simulink model "Foc_model_Matlab"  (R2024b)
settings: Solver=FixedStepDiscrete  StartTime=0.0  StopTime=5  FixedStep=Ts_simulink  RelTol=1e-3  EnableMultiTasking=on
PreLoadFcn:
  | mcb_pmsm_foc_hall_S32K144EVB_data;
InitFcn:
  | mbd_s32k_consistency_checks(bdroot(gcs));
model workspace (MAT data in the model file):
  IDC_OVERCURRENT : Simulink.Parameter (value not decoded)
  VDC_OVERVOLTAGE : Simulink.Parameter (value not decoded)
  VDC_UNDERVOLTAGE : Simulink.Parameter (value not decoded)
values from neighbouring files (symbols this model uses):
  epsilon_Id = 2    [Foc_data.m]
  epsilon_Iq = 90    [Foc_data.m]
  epsilon_w = 60    [Foc_data.m]
  K1 = 0.5    [Foc_data.m]
  K2 = 200    [Foc_data.m]
  Ki = 2500*Ts    (= 0.25)    [Foc_data.m]
  Kp = 70    [Foc_data.m]
  lambda_Id = 80    [Foc_data.m]
  lambda_Iq = 95    [Foc_data.m]
  lambda_w = 5    [Foc_data.m]
  rho_Id = 5    [Foc_data.m]
  rho_Iq = 55    [Foc_data.m]
  rho_w = 0.25    [Foc_data.m]
  Ts = T_pwm * 2    (= 0.0001)    [Foc_data.m]
  Ts_motor = T_pwm    (= 5e-05)    [Foc_data.m]
  Ts_simulink = T_pwm    (= 5e-05)    [Foc_data.m]
  Ts_speed = 10*Ts    (= 0.001)    [Foc_data.m]
undefined symbols (not defined in the file or in its folder): DiscIntNeverNeededParam, External, inverter, LQFP, mcb_isCodeGenVar, mcb_isSimVar, One, PI_params, pmsm, PU_System, Shot, sigbuilder_block, TRGMUX_PDB_TRIG
libraries: mbd_s32k1xx_ec_toolbox x39, mcbcontrolslib x9, simulink x7, mcbpositiondecoderlib x6, mbd_msd_ec_toolbox x5, hdlsllib x4, slpidlib x3, mcbhdlpositiondecoderlib x1, mcbplantlib x1, autolibpmsmexterior x1
(part 3 of 3)

== system Foc_model_Matlab/CurrentControl/Input Scaling/Read_Sensor (sim)/Subsystem ==
  Pos_Sim : Inport
  IIR Filter : mcbcontrolslib/IIR Filter  Commented=through  VariantControl=Low Pass Filter  VariantSelect=Low-pass  FilterConstantInputType=Specify via dialog  Filter_constant=0.01  advancedSettings=off  Ts=50e-6  cutOff_freq=32.1525
  Mechanical to Electrical Position : mcbpositiondecoderlib/Mechanical to Electrical Position  PolePairsInputType=Specify via dialog  NrPP=pmsm.p  selectedRange=Per unit  MechOfstInputType=Specify via dialog  mechOffsetIn=0  maxAngleIn=1  InputDataType=dataType  VariantSelect=floating-point
  Speed Measurement : mcbpositiondecoderlib/Speed Measurement  PositionUnit=Per unit  PositionScalingDatatype=uint32  SpeedCalculationMode=Time interval for speed calculation  SampleTimeAsync=Ts  MaximumApplicationSpeed=6000  SpeedResolution=5e-6  DelayLength=10  MaximumMeasurableSpeed=29999  MeasurableSpeedResolution=1.397e-05  SpeedUnit=Per unit based on dialog  PerUnitSpeed=pmsm.N_max  SpeedDataType=single
  Theta : Outport
  Speed : Outport  Port=2
  wires:
  Mechanical to Electrical Position/1 -> Theta/1
  Speed Measurement/1 -> IIR Filter/1
  Pos_Sim/1 -> Mechanical to Electrical Position/1, Speed Measurement/1
  IIR Filter/1 -> Speed/1

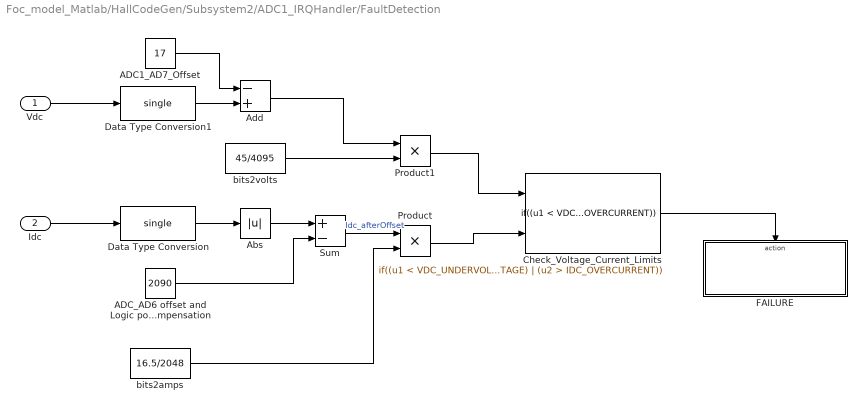
== system Foc_model_Matlab/HallCodeGen/Subsystem2/ADC1_IRQHandler/FaultDetection ==
  Vdc : Inport
  Idc : Inport  Port=2
  ADC1_AD7_Offset : Constant  Value=17  OutDataTypeStr=single
  ADC_AD6 offset and Logic power supply compensation : Constant  Value=2090  OutDataTypeStr=single
  Abs : Abs  SaturateOnIntegerOverflow=off
  Add : Sum  Inputs=-+  OutMin=0  OutMax=4095  OutDataTypeStr=single  AccumDataTypeStr=single  InputSameDT=on
  Check_Voltage_Current_Limits : If  NumInputs=2  IfExpression=(u1 < VDC_UNDERVOLTAGE) | (u1 > VDC_OVERVOLTAGE) | (u2 > IDC_OVERCURRENT)  ShowElse=off
  Data Type Conversion : DataTypeConversion  OutDataTypeStr=single  SaturateOnIntegerOverflow=off  RndMeth=Floor
  Data Type Conversion1 : DataTypeConversion  OutDataTypeStr=single  SaturateOnIntegerOverflow=off  RndMeth=Floor
  FAILURE : Subsystem  TreatAsAtomicUnit=on
  Product : Product  OutDataTypeStr=single
  Product1 : Product  OutDataTypeStr=single
  Sum : Sum  Inputs=+-  OutDataTypeStr=single  AccumDataTypeStr=single
  bits2amps : Constant  Value=16.5/2048  OutDataTypeStr=single
  bits2volts : Constant  Value=45/4095  OutDataTypeStr=single
  wires:
  Check_Voltage_Current_Limits/1 -> FAILURE/Action
  Idc/1 -> Data Type Conversion/1
  Data Type Conversion/1 -> Abs/1
  Vdc/1 -> Data Type Conversion1/1
  Abs/1 -> Sum/1
  ADC_AD6 offset and Logic power supply compensation/1 -> Sum/2
  Sum/1 -> Product/1  "Idc_afterOffset"
  Product/1 -> Check_Voltage_Current_Limits/2
  bits2amps/1 -> Product/2
  ADC1_AD7_Offset/1 -> Add/1
  Data Type Conversion1/1 -> Add/2
  bits2volts/1 -> Product1/2
  Add/1 -> Product1/1
  Product1/1 -> Check_Voltage_Current_Limits/1

== system Foc_model_Matlab/CurrentControl/Control_System/Current_Controllers/Controller_Id/Parametri_design ==
  Constant12 : Constant  Value=lambda_Id
  Constant13 : Constant  Value=epsilon_Id
  Constant2 : Constant  Value=rho_Id
  Data Store Read2 : DataStoreRead  DataStoreName=Lambda_d  IndexOptions=Index vector (dialog)  Indices=1  OutputSizes=1
  Data Store Read3 : DataStoreRead  DataStoreName=Epsilon_d  IndexOptions=Index vector (dialog)  Indices=1  OutputSizes=1
  Data Store Read4 : DataStoreRead  DataStoreName=Rho_d  IndexOptions=Index vector (dialog)  Indices=1  OutputSizes=1
  Mux1 : Mux  Inputs=3
  Mux2 : Mux  Inputs=3
  Variant Source3 : VariantSource
  Out1 : Outport
  wires:
  Constant13/1 -> Mux2/2
  Data Store Read3/1 -> Mux1/2
  Constant12/1 -> Mux2/1
  Constant2/1 -> Mux2/3
  Mux2/1 -> Variant Source3/2
  Mux1/1 -> Variant Source3/1
  Data Store Read2/1 -> Mux1/1
  Data Store Read4/1 -> Mux1/3
  Variant Source3/1 -> Out1/1

== system Foc_model_Matlab/CurrentControl/Control_System/Current_Controllers/Controller_Iq/Parametri_design ==
  Constant12 : Constant  Value=lambda_Iq
  Constant13 : Constant  Value=epsilon_Iq
  Constant2 : Constant  Value=rho_Iq
  Data Store Read2 : DataStoreRead  DataStoreName=Lambda_q  IndexOptions=Index vector (dialog)  Indices=1  OutputSizes=1
  Data Store Read3 : DataStoreRead  DataStoreName=Epsilon_q  IndexOptions=Index vector (dialog)  Indices=1  OutputSizes=1
  Data Store Read4 : DataStoreRead  DataStoreName=Rho_q  IndexOptions=Index vector (dialog)  Indices=1  OutputSizes=1
  Mux1 : Mux  Inputs=3
  Mux2 : Mux  Inputs=3
  Variant Source3 : VariantSource
  Out1 : Outport
  wires:
  Mux2/1 -> Variant Source3/2
  Constant12/1 -> Mux2/1
  Data Store Read3/1 -> Mux1/2
  Mux1/1 -> Variant Source3/1
  Constant13/1 -> Mux2/2
  Data Store Read2/1 -> Mux1/1
  Data Store Read4/1 -> Mux1/3
  Constant2/1 -> Mux2/3
  Variant Source3/1 -> Out1/1

== system Foc_model_Matlab/CurrentControl/Input Scaling/Read_Sensor (codegen)/Calculate Position from Hall/Atomic Hall Reading ==
  Data Store Read2 : DataStoreRead  DataStoreName=GlobalSpeedCount  IndexOptions=Index vector (dialog)  Indices=1  OutputSizes=1
  Data Store Read3 : DataStoreRead  DataStoreName=GlobalDirection  IndexOptions=Index vector (dialog)  Indices=1  OutputSizes=1
  Data Store Read4 : DataStoreRead  DataStoreName=GlobalSpeedValidity  IndexOptions=Index vector (dialog)  Indices=1  OutputSizes=1
  Data Store Read5 : DataStoreRead  Priority=1  DataStoreName=HallStateChangeFlag  IndexOptions=Index vector (dialog)  Indices=1  OutputSizes=1
  Hall Read : Subsystem
  Read_Register : mbd_s32k1xx_ec_toolbox/Utility Blocks/Read_Register  periph=ADC0  reg=SC1A  addr=0x4003B000  regSize=32  pcc_clock=ADC0_CLK
  HallState : Outport
  Count : Outport  Port=2
  SpeedCount : Outport  Port=3
  Dir : Outport  Port=4
  SpeedValidity : Outport  Port=5
  Hallchange : Outport  Port=6
  wires:
  Data Store Read4/1 -> SpeedValidity/1
  Data Store Read5/1 -> Hallchange/1
  Data Store Read2/1 -> SpeedCount/1
  Data Store Read3/1 -> Dir/1
  Hall Read/1(Out1) -> HallState/1
  Read_Register/1 -> Count/1

== system Foc_model_Matlab/HallCodeGen/Subsystem2/ADC1_IRQHandler/FaultDetection/FAILURE ==
  Action Port : ActionPort  ActionPortLabel=if((u1 < VDC_UNDERVOLTAGE) | (u1 > VDC_OVERVOLTAGE) | (u2 > IDC_OVERCURRENT))
  FAULT_read : DataStoreRead  DataStoreName=FAULT  IndexOptions=Index vector (dialog)  Indices=1  OutputSizes=1
  Failed Subsystem : Subsystem  TreatAsAtomicUnit=on
  If : If  IfExpression=u1 == 0  ShowElse=off
  wires:
  If/1 -> Failed Subsystem/Action
  FAULT_read/1 -> If/1

== system Foc_model_Matlab/CurrentControl/Input Scaling/Read_Sensor (codegen)/Calculate Position from Hall/Atomic Hall Reading/Hall Read ==
  Add1 : Sum  Inputs=+++  OutDataTypeStr=Inherit: Inherit via back propagation
  Bit Shift : hdlsllib/Logic and Bit Operations/Bit Shift  mode=Shift Left Logical  N=2
  Bit Shift1 : hdlsllib/Logic and Bit Operations/Bit Shift  mode=Shift Left Logical  N=1
  Data Type Conversion2 : DataTypeConversion  OutDataTypeStr=uint32  SaturateOnIntegerOverflow=off  RndMeth=Floor
  Data Type Conversion3 : DataTypeConversion  OutDataTypeStr=uint32  SaturateOnIntegerOverflow=off  RndMeth=Floor
  Data Type Conversion6 : DataTypeConversion  OutDataTypeStr=uint32  SaturateOnIntegerOverflow=off  RndMeth=Floor
  Digital_Input_HALL_A : mbd_s32k1xx_ec_toolbox/GPIO Blocks/Digital_Input  gpio_pin=PTD11: [PTD11 | Port D I/O]  pull_resistor=None  passive_filter=off
  Digital_Input_HALL_B : mbd_s32k1xx_ec_toolbox/GPIO Blocks/Digital_Input  gpio_pin=PTD10: [PTD10 | Port D I/O]  pull_resistor=None  passive_filter=off
  Digital_Input_HALL_C : mbd_s32k1xx_ec_toolbox/GPIO Blocks/Digital_Input  gpio_pin=PTA1: [PTA1 | Port A I/O]  pull_resistor=None  passive_filter=off
  Out1 : Outport
  wires:
  Add1/1 -> Out1/1
  Data Type Conversion2/1 -> Bit Shift1/1
  Bit Shift/1 -> Add1/1  "HALL_C_controller"
  Bit Shift1/1 -> Add1/2  "HALL_B_controller"
  Data Type Conversion6/1 -> Add1/3  "HALL_A_controller"
  Data Type Conversion3/1 -> Bit Shift/1
  Digital_Input_HALL_C/1 -> Data Type Conversion3/1
  Digital_Input_HALL_B/1 -> Data Type Conversion2/1
  Digital_Input_HALL_A/1 -> Data Type Conversion6/1

== system Foc_model_Matlab/HallCodeGen/Subsystem2/ADC1_IRQHandler/FaultDetection/FAILURE/Failed Subsystem ==
  Action Port : ActionPort  ActionPortLabel=if(u1 == 0)
  FAULT_write : DataStoreWrite  DataStoreName=FAULT  IndexOptions=Index vector (dialog)  Indices=1  OutputSizes=1
  FTM_PWM_Disable_Enable : mbd_s32k1xx_ec_toolbox/Motor Control Blocks/FTM Blocks/FTM_PWM_Disable_Enable  Priority=1  ftmModule=3  action=Disable
  NOK : Constant  OutDataTypeStr=boolean
  TPP_Functional_Mode : mbd_msd_ec_toolbox/TPP/TPP_Functional_Mode  tppInstance=0  action=Sleep
  wires:
  NOK/1 -> FAULT_write/1

== stateflow chart Foc_model_Matlab/Hardware Initialization/Enable PDB and start FTM ==
  settings: sampleTime=0.500
  state A
  state END
  (default) -> A
  A -> END : {enablePDB;}
  END -> END : {Normal_Op;}
  events: enablePDB output FUNCTION_CALL_EVENT; Normal_Op output FUNCTION_CALL_EVENT

== matlab function Foc_model_Matlab/CurrentControl/Control_System/Current_Controllers/Controller_Iq/MATLAB Function2 ==
  data: int_e_q input; reset output; info output; e_q input; Iq_fb input; Id_fb input; we input; Ld input; R input; Flux input; parameter input; limit input; V_ref output
function [reset, info, V_ref] = SMCq(int_e_q, e_q, Iq_fb, Id_fb, we, Ld, R, Flux, parameter, limit)
    lambda = parameter(1);
    epsilon = parameter(2);
    rho = parameter(3);
    % Inizializzazione variabili
    u_n = single(0);

  
    % Sliding Surface
    s = e_q + lambda*int_e_q;       

    %sat(s)
    if abs(s) > epsilon
        u_n = -rho*sign(s);
    else
        u_n = -rho*(s/epsilon);
    end

    % Legge di controllo
    u_eq = R*Iq_fb + Flux*we + Ld*(we*Id_fb - lambda*(e_q));
    V_ref_unsat = u_eq + u_n;
   

    % Applico la saturazione alla corrente di riferimento
    %sat(Te)
    if V_ref_unsat >= limit
        V_ref_unsat = limit;
        reset = single(1);
    elseif V_ref_unsat <= - limit
        V_ref_unsat = - limit;
        reset = single(1);
    else
        reset = single(0);
    end
    
    V_ref = V_ref_unsat;

    info = [u_eq, u_n, s, epsilon];

== matlab function Foc_model_Matlab/SpeedControl/Contrloller_wr/MATLAB Function ==
  data: reset output; info output; e_w input; int_e_w input; der_w_ref input; w_fb input; parameter input; J input; B input; Kt input; limit input; I_ref output
function [reset, info, I_ref] = SMCv(e_w, int_e_w, der_w_ref, w_fb, parameter, J, B, Kt, limit)

      
    % Inizializzazione variabili
    T_n = single(0);
    lambda = parameter(1);
    epsilon = parameter(2);
    rho = parameter(3);
    
    % Slinding Surface
    s = e_w + lambda*int_e_w;

    %sat(s)
    if abs(s) > epsilon
        T_n = - rho*sign(s);
    else
        T_n = - rho*(s/epsilon);
    end

    % Legge di controllo
    T_eq = B*w_fb + J*(der_w_ref - lambda*(e_w));
    
    % Legge di controllo
    T = T_eq + T_n;

    I_q_ref_unsat = single(T/Kt);   
    
    %sat(Te)
    if I_q_ref_unsat >= limit
        I_q_ref_unsat = limit;
        reset = single(1);
    elseif I_q_ref_unsat <= - limit
        I_q_ref_unsat = - limit;
        reset = single(1);
    else
        reset = single(0);
    end
    
    I_ref = I_q_ref_unsat;

    info = [T_eq, T_n, s, epsilon];

== matlab function Foc_model_Matlab/CurrentControl/Control_System/Current_Controllers/Controller_Id/MATLAB Function2 ==
  data: int_Id input; reset output; info output; Id_fb input; Iq_fb input; we input; parameter input; Lq input; R input; limit input; V_ref output
function [reset, info, V_ref] = SMCd(int_Id, Id_fb, Iq_fb, we, parameter, Lq, R, limit)

    % Inizializzazione variabili
    lambda = parameter(1);
    epsilon = parameter(2);
    rho = parameter(3);
    u_n = single(0);

    % Sliding Surface
    s = Id_fb + lambda*int_Id;       

    % Legge di controllo
    u_eq = R*Id_fb - Lq*(we*Iq_fb + lambda*(Id_fb));
    
    if abs(s) > epsilon
        u_n = -rho*sign(s);
    else
        u_n = -rho*(s/epsilon);
    end

    V_ref_unsat = u_eq + u_n;
   

    % Applico la saturazione alla corrente di riferimento
    %sat(Te)
    if V_ref_unsat >= limit
        V_ref_unsat = limit;
        reset = single(1);
    elseif V_ref_unsat <= - limit
        V_ref_unsat = - limit;
        reset = single(1);
    else
        reset = single(0);
    end
    
    V_ref = V_ref_unsat;

    info = [u_eq, u_n, s, epsilon];

== matlab function Foc_model_Matlab/CurrentControl/STSMO/Back-EMF Estimation ==
  data: v_alpha input; di_alpha_est output; di_beta_est output; e_alpha output; e_beta output; v_beta input; sat_ia input; sat_ib input; int_sat_ia input; int_sat_ib input; i_alpha_err input; i_beta_err input; i_alpha_est input; i_beta_est input; K1 input; K2 input
function [di_alpha_est, di_beta_est, e_alpha, e_beta]   = fcn(v_alpha, v_beta, sat_ia, sat_ib, int_sat_ia, int_sat_ib, i_alpha_err, i_beta_err, i_alpha_est, i_beta_est, K1, K2)


k1 = K1;
k2 = K2;         
R = 0.6367; %pmsm.Rs;
L = 0.000375; %pmsm.Ld;

z_alpha = k1*sqrt(abs(i_alpha_err))*sat_ia + k2*int_sat_ia;
z_beta = k1*sqrt(abs(i_beta_err))*sat_ib + k2*int_sat_ib;

di_alpha_est = -(R/L)*i_alpha_est + (1/L)*v_alpha - (1/L)*z_alpha;
di_beta_est = -(R/L)*i_beta_est + (1/L)*v_beta - (1/L)*z_beta;

e_alpha = z_alpha;
e_beta = z_beta;

== matlab function Foc_model_Matlab/CurrentControl/STSMO/Saturation  ==
  data: i_alpha input; sat_ia_error output; i_beta input; i_alpha_est input; i_beta_est input; sat_ib_error output; ia_error output; ib_error output; epsilona input; epsilonb input
function [sat_ia_error, sat_ib_error, ia_error, ib_error] = fcn( i_alpha, i_beta, i_alpha_est, i_beta_est, epsilona, epsilonb)

epsilon_a = epsilona;
epsilon_b = epsilonb;


ia_error = i_alpha_est - i_alpha;
ib_error = i_beta_est - i_beta;

if abs(ia_error) > epsilon_a
    sat_ia_error = sign(ia_error);
else
    sat_ia_error = abs(ia_error) / epsilon_a;
end

if abs(ib_error) > epsilon_b
    sat_ib_error = sign(ib_error);
else
    sat_ib_error = abs(ib_error) / epsilon_b;
end
